simulink model "Tarea4_Luminosidad3CanalesRGB"  (R2022b)
settings: Solver=VariableStepAuto  StartTime=0.0  StopTime=10.0  RelTol=1e-3
undefined symbols (not defined in the file): concatena1, gray, none, videoinput
libraries: visionstatistics x3, visiontextngfix x3, visionconversions x3, imaqlib x1, visionsources x1
settings Model: Creator=esteb  LastModifiedBy=esteb

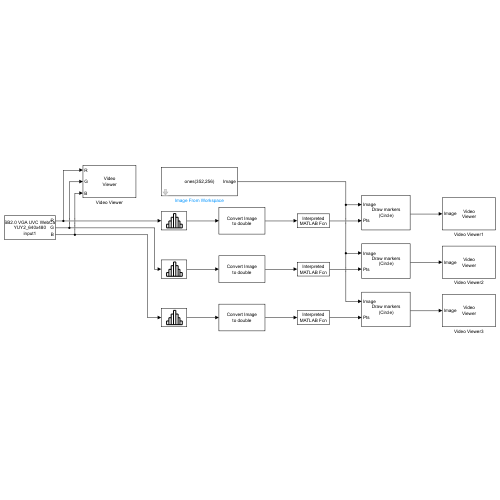
[thumbnail: Simulink's stored preview of the top-level diagram]
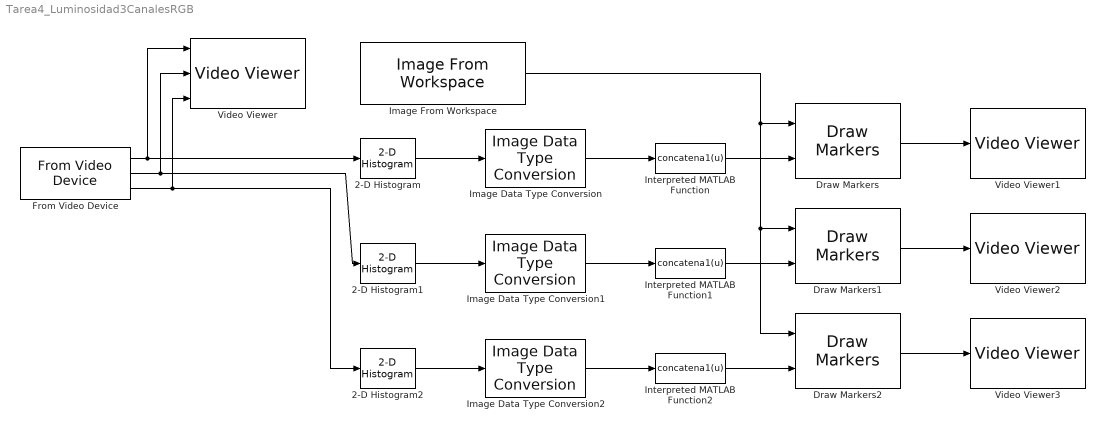
== system Tarea4_Luminosidad3CanalesRGB ==
  2-D Histogram : visionstatistics/2-D Histogram  umin=0  umax=1  nbins=256  operateOver=Entire input  normalized=on  run=off  reset=on  trigtype=None  Dimension=1  colComp=on  roundingMode=Floor  overflowMode=off
  2-D Histogram1 : visionstatistics/2-D Histogram  umin=0  umax=1  nbins=256  operateOver=Entire input  normalized=on  run=off  reset=on  trigtype=None  Dimension=1  colComp=on  roundingMode=Floor  overflowMode=off
  2-D Histogram2 : visionstatistics/2-D Histogram  umin=0  umax=1  nbins=256  operateOver=Entire input  normalized=on  run=off  reset=on  trigtype=None  Dimension=1  colComp=on  roundingMode=Floor  overflowMode=off
  Draw Markers : visiontextngfix/Draw Markers  shape=Circle  size=3  fill=off  fillClrSource=Specify via dialog  display=Black  intensity=200  color=[200 255 100]  opacity=0.6  viewport=Entire image  antialiasing=off  inType=Obsolete  imagePorts=One multidimensional signal  roundingMode=Floor  overflowMode=off  memoryMode=Specify word length  memoryWordLength=16  memoryFracLength=15  prodOutputMode=Binary point scaling  prodOutputWordLength=32  prodOutputFracLength=14
  Draw Markers1 : visiontextngfix/Draw Markers  shape=Circle  size=3  fill=off  fillClrSource=Specify via dialog  display=Black  intensity=200  color=[200 255 100]  opacity=0.6  viewport=Entire image  antialiasing=off  inType=Obsolete  imagePorts=One multidimensional signal  roundingMode=Floor  overflowMode=off  memoryMode=Specify word length  memoryWordLength=16  memoryFracLength=15  prodOutputMode=Binary point scaling  prodOutputWordLength=32  prodOutputFracLength=14
  Draw Markers2 : visiontextngfix/Draw Markers  shape=Circle  size=3  fill=off  fillClrSource=Specify via dialog  display=Black  intensity=200  color=[200 255 100]  opacity=0.6  viewport=Entire image  antialiasing=off  inType=Obsolete  imagePorts=One multidimensional signal  roundingMode=Floor  overflowMode=off  memoryMode=Specify word length  memoryWordLength=16  memoryFracLength=15  prodOutputMode=Binary point scaling  prodOutputWordLength=32  prodOutputFracLength=14
  From Video Device : imaqlib/From Video Device  DeviceMenu=winvideo 1 (USB2.0 VGA UVC WebCam)  Device=winvideo 1 (USB2.0 VGA UVC WebCam)  ObjConstructor=videoinput('winvideo', 1)  VideoFormatMenu=YUY2_640x480  VideoFormat=YUY2_640x480  VideoSource=input1  ROIPosition=[0 0 480 640]  EnableHWTrigger=off  TriggerConfiguration=none/none  SampleTime=1/30  OutputPortsMode=Separate color signals  DataType=single  CanDoHWTrigger=no  ReturnedColorSpace=rgb  BlockHandle=4.0002  ROIWidth=640  ROIHeight=480  ROIColumn=0  ROIRow=0  EngXMLPath=C:\Program Files\MATLAB\R2022b\toolbox\imaq\imaq\private  DevXMLPath=C:\ProgramData\MATLAB\SupportPackages\R2022b\toolbox\imaq\supportpackages\genericvideo\adaptor\win64  EngLibPath=C:\Program Files\MATLAB\R2022b\toolbox\imaq\imaqblks\imaqmex\win64  ColorSpace=rgb  BayerSensorAlignment=grbg  ImaqMode=off
  Image Data Type Conversion : visionconversions/Image Data Type Conversion  outDT=double  isSigned=on  wordLen=16  numFracBits=0
  Image Data Type Conversion1 : visionconversions/Image Data Type Conversion  outDT=double  isSigned=on  wordLen=16  numFracBits=0
  Image Data Type Conversion2 : visionconversions/Image Data Type Conversion  outDT=double  isSigned=on  wordLen=16  numFracBits=0
  Image From Workspace : visionsources/Image From Workspace  Tag=vipblks_nd  ImageValue=ones(352,256)  Ts=inf  imagePorts=One multidimensional signal  OutPortLabels=R|G|B  ImageDataType=Inherit from 'Value'  Signed=on  WordLength=16  sdImageDataType=sfix(16)  FractionLengthMode=User-defined  FractionLength=15
  Interpreted MATLAB Function : MATLABFcn  MATLABFcn=concatena1(u)  Output1D=off
  Interpreted MATLAB Function1 : MATLABFcn  MATLABFcn=concatena1(u)  Output1D=off
  Interpreted MATLAB Function2 : MATLABFcn  MATLABFcn=concatena1(u)  Output1D=off
  Video Viewer : VideoViewer  imagePorts=separate color signals  FigPos=[559 583 418 304]
  Video Viewer1 : VideoViewer  colormapValue=gray(256)  FigPos=[154.6 701.2 417.6 304]
  Video Viewer2 : VideoViewer  FigPos=[784.2 621.2 417.6 304]
  Video Viewer3 : VideoViewer  FigPos=[925 728.4 417.6 304]
  wires:
  Image Data Type Conversion/1 -> Interpreted MATLAB Function/1
  Interpreted MATLAB Function/1 -> Draw Markers/2
  Image From Workspace/1 -> Draw Markers2/1, Draw Markers1/1, Draw Markers/1
  Draw Markers/1 -> Video Viewer1/1
  From Video Device/1 -> 2-D Histogram/1, Video Viewer/1
  From Video Device/2 -> Video Viewer/2, 2-D Histogram1/1
  From Video Device/3 -> 2-D Histogram2/1, Video Viewer/3
  2-D Histogram/1 -> Image Data Type Conversion/1
  2-D Histogram1/1 -> Image Data Type Conversion1/1
  Image Data Type Conversion1/1 -> Interpreted MATLAB Function1/1
  2-D Histogram2/1 -> Image Data Type Conversion2/1
  Image Data Type Conversion2/1 -> Interpreted MATLAB Function2/1
  Interpreted MATLAB Function1/1 -> Draw Markers1/2
  Interpreted MATLAB Function2/1 -> Draw Markers2/2
  Draw Markers1/1 -> Video Viewer2/1
  Draw Markers2/1 -> Video Viewer3/1
